simulink model "pulsegen"  (Simulink 7.8)
settings: Solver=ode45  StartTime=0.0  StopTime=2000.0  RelTol=1e-3
undefined symbols (not defined in the file or in its folder): inRate, shift
settings Model: Creator=Leo  LastModifiedBy=Leo

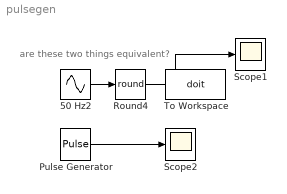
== system pulsegen ==
  note: are these two things equivalent?
  50 Hz2 : Sin  Amplitude=0.5  Bias=inRate/20000  Frequency=(inRate*2*pi)/1000  Phase=-shift*100/(2*pi*inRate)  SampleTime=0
  Pulse Generator : DiscretePulseGenerator  PulseType=Time based  Period=inRate*10*pi  PhaseDelay=shift
  Round4 : Rounding  Operator=round
  Scope1 : Scope
  Scope2 : Scope
  To Workspace : ToWorkspace  VariableName=doit  SampleTime=-1  SaveFormat=Array
  wires:
  50 Hz2/1 -> Round4/1
  Pulse Generator/1 -> Scope2/1
  Round4/1 -> To Workspace/1, Scope1/1
